simulink model "Problem2"  (R2020b)
settings: Solver=VariableStepAuto  StartTime=0.0  StopTime=100  RelTol=1e-3
PreLoadFcn:
  | load('data.mat')
InitFcn:
  | t = [1:100]';
model workspace (MAT data in the model file):
  b = 50
  k1 = 25
  k2 = 50
  m1 = 100
  m2 = 20
  road = [0 0 0 1 1 1 1 0 0 0]
settings Model: Creator=Acer  LastModifiedBy=Acer
settings DataIOCC: ExternalInput=[t, bumpyroad]  LoadExternalInput=on  SaveFormat=Array  SaveOutput=off  SignalLogging=off  DSMLogging=off  SaveTime=off  ReturnWorkspaceOutputs=off

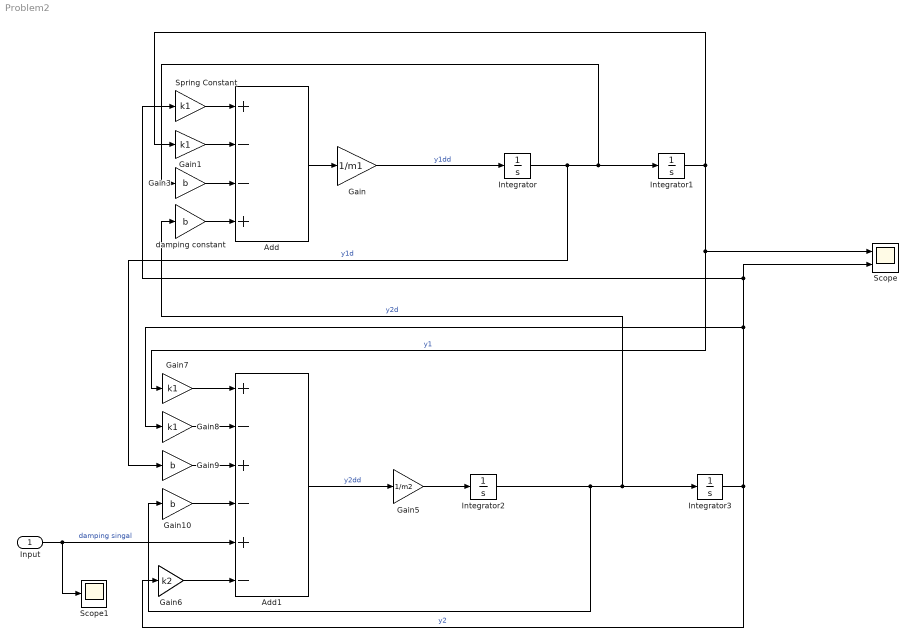
== system Problem2 ==
  Input : Inport
  Add : Sum  Inputs=+--+
  Add1 : Sum  Inputs=+-+-+-
  Gain : Gain  Gain=1/m1
  Gain1 : Gain  Gain=k1
  Gain10 : Gain  Gain=b
  Gain3 : Gain  Gain=b
  Gain5 : Gain  Gain=1/m2
  Gain6 : Gain  Gain=k2
  Gain7 : Gain  Gain=k1
  Gain8 : Gain  Gain=k1
  Gain9 : Gain  Gain=b
  Integrator{,1..3} (4 alike) : Integrator
  Scope : Scope  NumInputPorts=2
  Scope1 : Scope
  Spring Constant : Gain  Gain=k1
  damping constant : Gain  Gain=b
  wires:
  Integrator/1 -> Gain9/1, Gain3/1, Integrator1/1  "y1d"
  Integrator2/1 -> Gain10/1, Integrator3/1, damping constant/1  "y2d"
  Integrator3/1 -> Gain6/1, Gain8/1, Scope/2, Spring Constant/1  "y2"
  Gain/1 -> Integrator/1  "y1dd"
  Integrator1/1 -> Gain1/1, Gain7/1, Scope/1  "y1"
  Add/1 -> Gain/1
  Gain1/1 -> Add/2
  Spring Constant/1 -> Add/1
  Gain3/1 -> Add/3
  damping constant/1 -> Add/4
  Add1/1 -> Gain5/1  "y2dd"
  Gain5/1 -> Integrator2/1
  Gain6/1 -> Add1/6
  Gain7/1 -> Add1/1
  Gain8/1 -> Add1/2
  Gain9/1 -> Add1/3
  Gain10/1 -> Add1/4
  Input/1 -> Scope1/1, Add1/5  "damping singal"
